simulink model "LabeledDefaultTransition"  (R2020b)
settings: Solver=VariableStepAuto  StartTime=0.0  StopTime=10.0  RelTol=1e-3
settings Model: Creator=apple  LastModifiedBy=apple

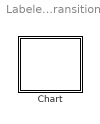
== system LabeledDefaultTransition ==
  Chart : Stateflow chart  TreatAsAtomicUnit=on

== stateflow chart LabeledDefaultTransition/Chart ==
  state A
    en:fprintf("Entry A");
    du:fprintf("During A");
    ex:fprintf("Exit A");
  state B
    en:fprintf("Entry B");
    du:fprintf("During B");
    ex:fprintf("Exit B");
    state B1
      en:fprintf("Entry B1");
    state B2
      en:fprintf("Entry B2");
    (default) -> B1 [order 1] : E_one
    (default) -> B2 [order 2]
  (default) -> A
  A -> B : E_one || E_two
  events: E_one local FUNCTION_CALL_EVENT; E_two local FUNCTION_CALL_EVENT
